simulink model "EEE3099S_LineFollowStateflowSim"  (R2021b)
settings: Solver=FixedStepDiscrete  StartTime=0.0  StopTime=30  FixedStep=0.01  RelTol=1e-3
undefined symbols (not defined in the file or in its folder): InputPWM, WheelSpeed
libraries: mobileRoboticsTrainingLib x5
settings Model: Creator=Boitumelo  LastModifiedBy=gamin

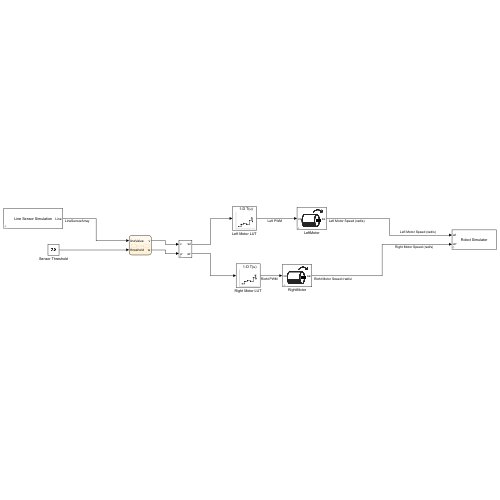
[thumbnail: Simulink's stored preview of the top-level diagram]
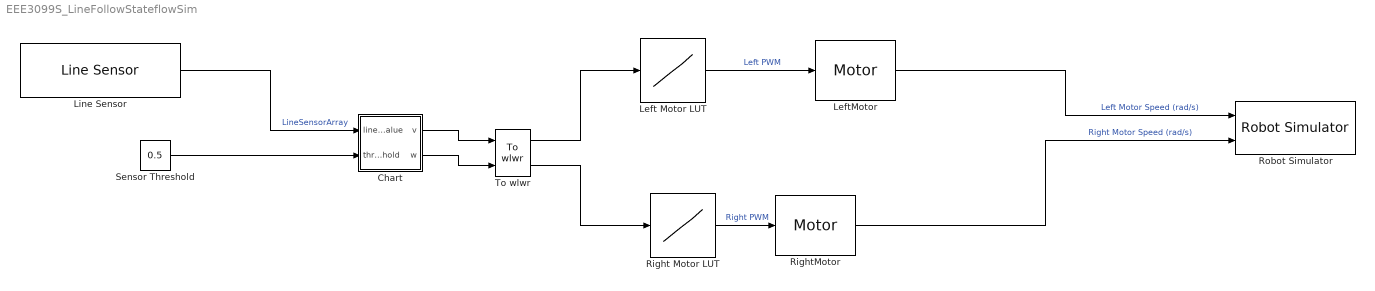
== system EEE3099S_LineFollowStateflowSim ==
  Chart : Stateflow chart  TreatAsAtomicUnit=on
  Left Motor LUT : Lookup_n-D  NumberOfTableDimensions=1  BreakpointsForDimension1=WheelSpeed  Table=InputPWM  InterpMethod=Nearest  ExtrapMethod=Clip  InternalRulePriority=Speed  RndMeth=Simplest  InputSameDT=on
  LeftMotor : mobileRoboticsTrainingLib/Motor  motorPlant=wheelMotorModel  sensorType=Speed
      settings: SourceProductName=Mobile Robotics Training Library
  Line Sensor : mobileRoboticsTrainingLib/Line Sensor  mapVariable=mapForSim  envVal=1  lineVal=0  sensOff=[0.01 0]
      settings: SourceProductName=Mobile Robotics Training Library
  Right Motor LUT : Lookup_n-D  NumberOfTableDimensions=1  BreakpointsForDimension1=WheelSpeed  Table=InputPWM  InterpMethod=Nearest  ExtrapMethod=Clip  InternalRulePriority=Speed  RndMeth=Simplest  InputSameDT=on
  RightMotor : mobileRoboticsTrainingLib/Motor  motorPlant=wheelMotorModel  sensorType=Speed
      settings: SourceProductName=Mobile Robotics Training Library
  Robot Simulator : mobileRoboticsTrainingLib/Robot Simulator  Priority=99  mapVar=mapForSim  startX=0.48557  startY=0.11149  startTheta=90  axleLength=axleLength  wheelR=wheelR
  Sensor Threshold : Constant  Value=0.5
  To wlwr : mobileRoboticsTrainingLib/To wlwr  axleLength=axleLength  wheelR=wheelR
  wires:
  Right Motor LUT/1 -> RightMotor/1  "Right PWM"
  Left Motor LUT/1 -> LeftMotor/1  "Left PWM"
  To wlwr/1 -> Left Motor LUT/1
  To wlwr/2 -> Right Motor LUT/1
  Line Sensor/1 -> Chart/1(lineValue)  "LineSensorArray"
  RightMotor/1 -> Robot Simulator/2  "Right Motor Speed (rad/s)"
  LeftMotor/1 -> Robot Simulator/1  "Left Motor Speed (rad/s)"
  Sensor Threshold/1 -> Chart/2(threshold)
  Chart/2(w) -> To wlwr/2
  Chart/1(v) -> To wlwr/1

== stateflow chart EEE3099S_LineFollowStateflowSim/Chart ==
  state goLeft
    v = 0.5
    w = 7
  state goRight
    v = 0.5
    w = -7
  (default) -> goLeft
  goRight -> goLeft : [lineValue<threshold]
  goLeft -> goRight : [lineValue>=threshold]
  data: lineValue input; threshold input; v output; w output
